simulink model "IIR_Filter_int32"  (Simulink 8.2)
settings: Solver=FixedStepDiscrete  StartTime=0.0  StopTime=10.0  FixedStep=0.001  RelTol=1e-3
settings Model: Creator=reynaudp  LastModifiedBy=reynaudp  SimulationMode=processor-in-the-loop (pil)
settings DataIOCC: SignalLoggingSaveFormat=Dataset
settings OptimizationCC: InlineParams=on  OptimizeModelRefInitCode=on  LifeSpan=1
settings DebuggingCC: FcnCallInpInsideContextMsg=EnableAllAsError  ModelReferenceSymbolNameMessage=none
settings HardwareCC: ProdLargestAtomicInteger=Integer  ProdLargestAtomicFloat=Float  ProdIntDivRoundTo=Zero  ProdEndianess=LittleEndian  ProdHWDeviceType=STMicroelectronics->STM32F4xx 32-bit Cortex-M4
settings ModelReferenceCC: SupportModelReferenceSimTargetCustomCode=on
settings RTWCC: SystemTargetFile=stm32F4xx.tlc  TemplateMakefile=stm32F4xx.tmf  Description=stm32F4xx (Embedded Target)  GenerateReport=on  ProcessScript=stm32F4xx_make_rtw_hook  IncludeHyperlinkInReport=on  LaunchReport=on  GenerateCodeReplacementReport=on
settings CodeAppCC: IgnoreCustomStorageClasses=off  CustomSymbolStrType=$N$R$M  InternalIdentifier=Classic
settings STFCustomTargetCC: CodeReplacementLibrary=ANSI_C  ParMdlRefBuildCompliant=on  IncludeMdlTerminateFcn=off  CombineOutputUpdateFcns=on  ERTCustomFileBanners=on  SupportContinuousTime=off  SupportNonInlinedSFcns=off  MATLABClassNameForMDSCustomization=Simulink.SoftwareTarget.ERTCustomization  GRTInterface=off  SystemTargetFile=stm32F4xx.tlc
settings ERTTargetCC: CodeReplacementLibrary=ANSI_C  MultiwordLength=2048  CompOptLevelCompliant=off  ConcurrentExecutionCompliant=off  IncludeMdlTerminateFcn=off  ERTFirstTimeCompliant=off  ModelStepFunctionPrototypeControlCompliant=off  CPPClassGenCompliant=off  InlinedParameterPlacement=NonHierarchical  ERTSrcFileBannerTemplate=sourceFileTemplate.cgt  ERTHdrFileBannerTemplate=sourceFileTemplate.cgt  ERTDataSrcFileTemplate=sourceFileTemplate.cgt  ERTDataHdrFileTemplate=sourceFileTemplate.cgt  ERTCustomFileTemplate=customRoutineProcess.tlc  ConvertIfToSwitch=off  SuppressUnreachableDefaultCases=off
settings CustomProperty: DataType=RTWOptions_EnumType_C__Matlab_STM32F4xx_rtw_stm32F4xx_1stm32Target  Value=STM32F4xxx
settings EnumStrPairs: String=STM32F4xxx

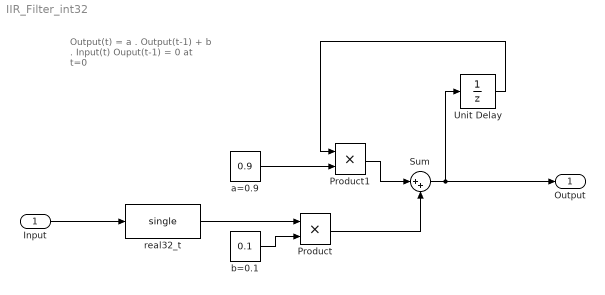
== system IIR_Filter_int32 ==
  note: Output(t) = a . Output(t-1) + b . Input(t)
      | Ouput(t-1) = 0 at t=0
  Input : Inport  OutDataTypeStr=int32
  Product : Product  RndMeth=Zero  OutDataTypeStr=Inherit: Same as first input
  Product1 : Product  RndMeth=Zero  OutDataTypeStr=Inherit: Same as first input
  Sum : Sum  Inputs=|++  OutDataTypeStr=Inherit: Same as first input
  Unit Delay : UnitDelay  SampleTime=-1
  a=0.9 : Constant  Value=0.9  VectorParams1D=off  OutDataTypeStr=single
  b=0.1 : Constant  Value=0.1  OutDataTypeStr=single  LockScale=on
  real32_t : DataTypeConversion  OutDataTypeStr=single
  Output : Outport  OutDataTypeStr=single
  wires:
  Input/1 -> real32_t/1
  Unit Delay/1 -> Product1/1
  Product1/1 -> Sum/1
  Product/1 -> Sum/2
  b=0.1/1 -> Product/2
  a=0.9/1 -> Product1/2
  real32_t/1 -> Product/1
  Sum/1 -> Unit Delay/1, Output/1
